simulink subsystem "OdometriaZ"  (R2025a)
settings: Solver=VariableStepAuto  StartTime=0.0  StopTime=10.0  RelTol=1e-3
undefined symbols (not defined in the file): DiscIntNeverNeededParam
settings Model: Creator=Antonio  LastModifiedBy=aj
settings RTWCC: GPUComputeCapability=3.5

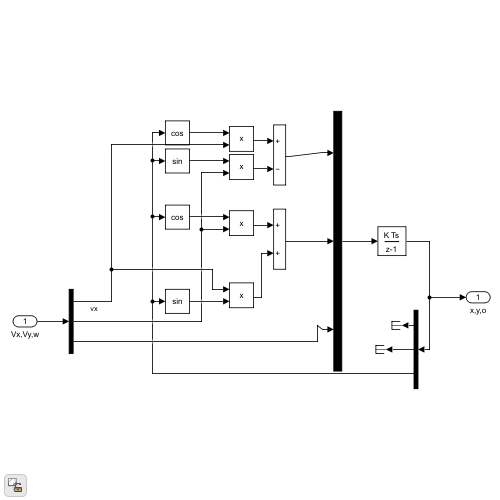
[thumbnail: Simulink's stored preview of the top-level diagram]
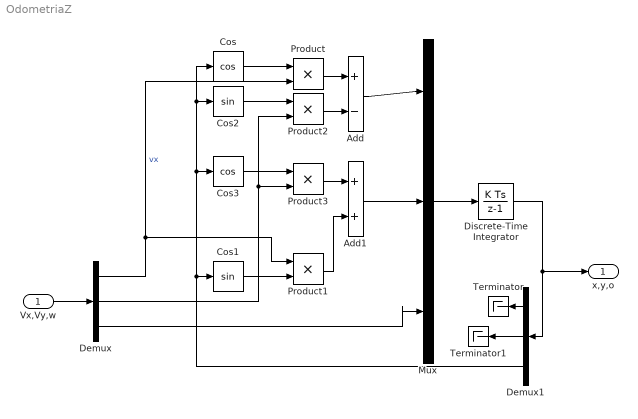
== system OdometriaZ ==
  Vx,Vy,w : Inport
  Add : Sum  Inputs=+-
  Add1 : Sum
  Cos : Trigonometry  Operator=cos
  Cos1 : Trigonometry
  Cos2 : Trigonometry
  Cos3 : Trigonometry  Operator=cos
  Demux : Demux  Outputs=3
  Demux1 : Demux  Outputs=3
  Discrete-Time Integrator : DiscreteIntegrator  SampleTime=-1  ICPrevOutput=DiscIntNeverNeededParam  ICPrevScaledInput=DiscIntNeverNeededParam
  Mux : Mux  Inputs=3
  Product{,1..3} (4 alike) : Product
  Terminator : Terminator
  Terminator1 : Terminator
  x,y,o : Outport
  wires:
  Vx,Vy,w/1 -> Demux/1
  Cos/1 -> Product/1
  Cos1/1 -> Product1/2
  Discrete-Time Integrator/1 -> x,y,o/1, Demux1/1
  Mux/1 -> Discrete-Time Integrator/1
  Product/1 -> Add/1
  Product1/1 -> Add1/2
  Demux/3 -> Mux/3
  Demux1/3 -> Cos/1, Cos2/1, Cos3/1, Cos1/1
  Demux/1 -> Product/2, Product1/1  "vx"
  Demux1/1 -> Terminator/1
  Demux1/2 -> Terminator1/1
  Product2/1 -> Add/2
  Cos2/1 -> Product2/1
  Demux/2 -> Product2/2, Product3/2
  Add/1 -> Mux/1
  Product3/1 -> Add1/1
  Cos3/1 -> Product3/1
  Add1/1 -> Mux/2
